simulink model "p8"  (R2017b)
settings: Solver=VariableStepAuto  StartTime=0.0  StopTime=10.0  RelTol=1e-3
settings Model: Creator=Rita Monteiro  LastModifiedBy=Rita Monteiro

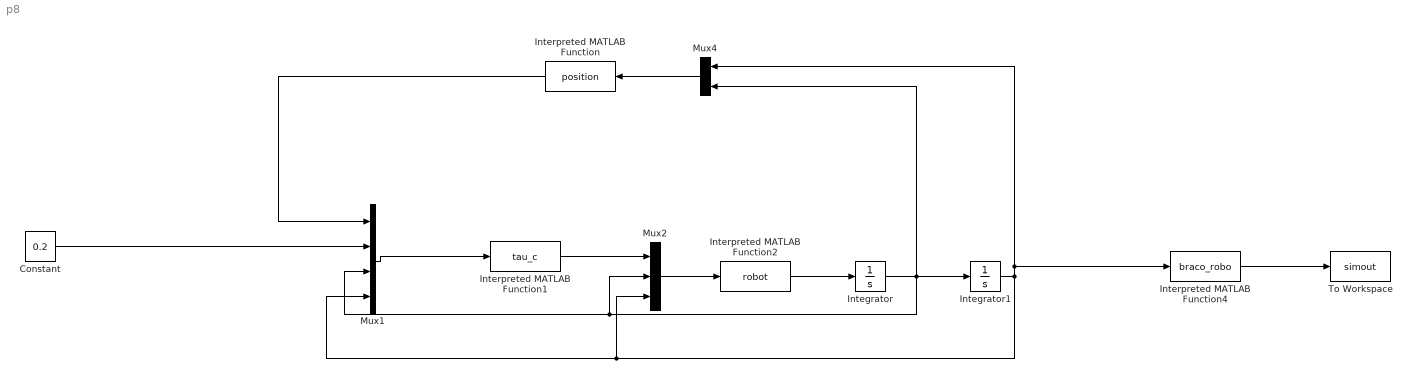
== system p8 ==
  Constant : Constant  Value=0.2
  Integrator : Integrator  InitialCondition=[0;0]
  Integrator1 : Integrator  InitialCondition=[pi/2;pi/4]
  Interpreted MATLAB Function : MATLABFcn  MATLABFcn=position
  Interpreted MATLAB Function1 : MATLABFcn  MATLABFcn=tau_c
  Interpreted MATLAB Function2 : MATLABFcn  MATLABFcn=robot
  Interpreted MATLAB Function4 : MATLABFcn  MATLABFcn=braco_robo  OutputDimensions=1
  Mux1 : Mux
  Mux2 : Mux  Inputs=3
  Mux4 : Mux  Inputs=2
  To Workspace : ToWorkspace  VariableName=simout  SampleTime=-1
  wires:
  Constant/1 -> Mux1/2
  Interpreted MATLAB Function/1 -> Mux1/1
  Mux1/1 -> Interpreted MATLAB Function1/1
  Interpreted MATLAB Function1/1 -> Mux2/1
  Mux2/1 -> Interpreted MATLAB Function2/1
  Interpreted MATLAB Function2/1 -> Integrator/1
  Integrator1/1 -> Interpreted MATLAB Function4/1, Mux4/1, Mux1/4, Mux2/3
  Interpreted MATLAB Function4/1 -> To Workspace/1
  Mux4/1 -> Interpreted MATLAB Function/1
  Integrator/1 -> Mux4/2, Integrator1/1, Mux1/3, Mux2/2
